simulink model "W1Q3"  (R2020a)
settings: Solver=VariableStepAuto  StartTime=0.0  StopTime=1  RelTol=1e-3
values from neighbouring files (symbols this model uses):
  noise = 2*pi*100    (= 628.318530718)    [para.m]
  signal = 2*pi*1000    (= 6283.18530718)    [para.m]
settings Model: Creator=Vinayak  LastModifiedBy=Vinayak

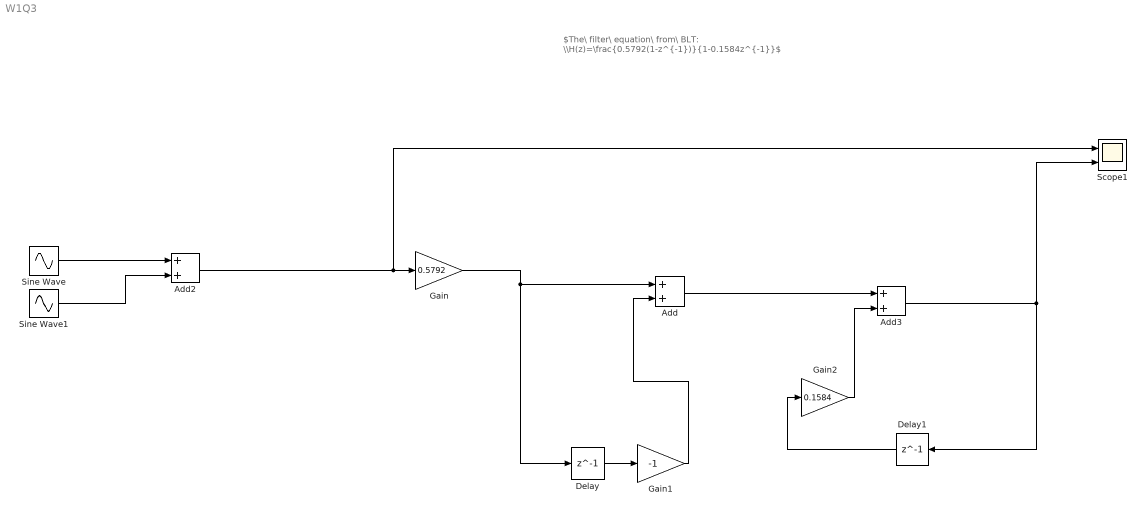
== system W1Q3 ==
  note: $The\ filter\ equation\ from\ BLT: \\H(z)=\frac{0.5792(1-z^{-1})}{1-0.1584z^{-1}}$
  Add : Sum
  Add2 : Sum
  Add3 : Sum
  Delay : Delay  DelayLength=1
  Delay1 : Delay  DelayLength=1
  Gain : Gain  Gain=0.5792
  Gain1 : Gain  Gain=-1
  Gain2 : Gain  Gain=0.1584
  Scope1 : Scope  NumInputPorts=2
  Sine Wave : Sin  Frequency=noise  SampleTime=0
  Sine Wave1 : Sin  Frequency=signal  SampleTime=0
  wires:
  Delay/1 -> Gain1/1
  Gain/1 -> Delay/1, Add/1
  Sine Wave1/1 -> Add2/2
  Add2/1 -> Scope1/1, Gain/1
  Gain1/1 -> Add/2
  Sine Wave/1 -> Add2/1
  Delay1/1 -> Gain2/1
  Add3/1 -> Scope1/2, Delay1/1
  Gain2/1 -> Add3/2
  Add/1 -> Add3/1
